simulink model "bike_model_yixiao"  (R2018b)
settings: Solver=FixedStepAuto  StartTime=0.0  StopTime=sim_time  FixedStep=Ts_IMU  MaxStep=Ts  RelTol=1e-3
undefined symbols (not defined in the file): A, A_kalman, B, b_compFilter, B_kalman, b_real, C, C_kalman, complementary, cumulative_dist_along_path, curvature, D, D_kalman, damp, Dead_Band, delay, direct_control, DiscIntNeverNeededParam, Discrete, DX, filter_model, forward_motor_dynamics, fr_oscil, g, gain, I_direct, I_lat, I_steer, IMU_height_model, IMU_height_real, initial_states, initial_x, initial_y, input_velocity, lambda_compFilter, lambda_real, lat_control, look_ahead, lqr_gains, max_handlebar, max_roll, max_steering_motor_acc, max_steering_motor_speed, min_handlebar, min_roll, min_steering_motor_acc, min_steering_motor_speed, Nc, noise, noise_acc, noise_encoder, noise_gyro, noise_hall, noise_pos_meas, Np, osc_roll, osc_steer, P_direct, P_lat, P_steer ... (+20)
libraries: simulink x14, mpclib x2, dspsigops x2, simulink_extras x1, ctrlSharedLib x1
(part 3 of 3)

== matlab function bike_model_yixiao/Balance Controller/MPC attempt 2/MATLAB Function3 ==
  data: x0 input; u output; eta output; xk0 input size=6; u0 input; Nc input; Np input; r input; Delta_t input; xk output size=6; v input
function [u,eta,xk] =  mpc_setpointcontrol(x0,xk0,u0,Nc,Np,r,Delta_t,v)
    coder.extrinsic('mpc_setpoint')
    [u,eta,xk] =  mpc_setpoint(x0,xk0,u0,Nc,Np,r,Delta_t,v);
end

== matlab function bike_model_yixiao/Global Angles and Coordinates Calculator - Velocity/Measured Global Angles to Global Coordinates/MATLAB Function1 ==
  data: v input; psi input; Xdot output; beta input; Ydot output
function [Xdot, Ydot]  = fcn(v, psi, beta)

Xdot = v * cos(psi + beta);
Ydot = v * sin(psi + beta);

== matlab function bike_model_yixiao/Physical Bike/Global Angles and Coordinates Calculator - Position/Measured Global Angles to Global Coordinates/MATLAB Function1 ==
  data: v input; psi input; Xdot output; beta input; Ydot output
function [Xdot, Ydot]  = fcn(v, psi, beta)

Xdot = v * cos(psi + beta);
Ydot = v * sin(psi + beta);
